simulink model "CAVE_MachE_dSPACE_250912"  (R2024a)
settings: configuration reference "ConfigSetDesktopFixedStep" (kept outside this file)
PreLoadFcn:
  | VSS_BICYCLE=Simulink.Variant('Dual=0');
  | VSS_DUAL=Simulink.Variant('Dual=1');
  | Dual=1;
  | load('DriveCycle2.mat')
PostLoadFcn:
  | if any(exist('dsrtsu_mdlpostloadfcn', 'file') ~= 0), dsrtsu_mdlpostloadfcn('Execute', bdroot); end
InitFcn:
  | , if any(exist('rtifpga_mdlclblib', 'file') ~= 0), rtifpga_mdlclblib('Init', bdroot); end,
  | , if any(exist('dsmpb_private', 'file') ~= 0), dsmpb_private('dsmpb_mdlclblib', 'Init', bdroot); end,
  | load('DriveCycle2.mat')
model workspace (MAT data in the model file):
  Gas = 0.383333333333
values from neighbouring files (symbols this model uses):
  CoastDown =     [Run_Simulink.mat]
  limitedMCT =     [Run_Simulink.mat]
  MCT =     [Run_Simulink.mat]
  pMCT =     [Run_Simulink.mat]
  RealSimPara =     [Run_Simulink.mat]
  Ref_speed = [13 13.007895099 13.015778396 13.023649891 13.031509584 13.039357475 13.047193564 13.055017851 13.062830336 13.070631019 13.0784199 13.086196979 ... (2669 elements, 2669x1)]    [Ref_speed_and_time.mat]
  Ref_time = [0 0.01 0.02 0.03 0.04 0.05 0.06 0.07 0.08 0.09 0.1 0.11 ... (2669 elements, 2669x1)]    [Ref_speed_and_time.mat]
  US06 =     [Run_Simulink.mat]
undefined symbols (not defined in the file or in its folder): AccelCmd, ActTqLF_Nm_, ActTqLR_Nm_, ActTqRF_Nm_, ActTqRR_Nm_, BattChargeLimitMaxPwr, BattChargeLimitSocBpts, BattChargeLimitTbl, BattChrgCapcty, BattDischargeLimitSocBpts, BattDischargeLimitTbl, BattDischargeMaxPwr, BattNumCellsParallel, BattNumCellsSeries, BattOpenVoltCapBpts, BattOpenVoltTbl, BattResistSocBpts, BattResistTbl, BattResistTempBpts, BrakeMaxPrs, BrakeMaxTrq, ChassisDistCg2FrontAxle, ChassisDistCg2RearAxle, ChassisVehMass, CltchCmd, DecelCmd, DiffRatio, DiscIntNeverNeededParam, EnvGravCnst, EnvPrs, EnvTemp, FuelSpecificGrav, GearCmd, h, InitStates, lgSw, MtrEffSpdBpts, MtrEffTbl, MtrEffTrqBpts, MtrPwrMax, MtrTrqMax, SteeringCmd, SupvsryCtrlRegenBrkCutOffTbl, SupvsryCtrlRegenSpdBpts, TestScnrioCycleNum, VEH
libraries: VSIGenLib x122, simulink x112, etargetslib x75, dsmpblib x55, vehdynlibtire x24, CarMaker4SL x20, autolibshared x19, vehdynlibsuspension x14, vehdynlibtirecommon x14, autolibutils x10, VsrLibWheel x8, autolibpowerinfoutils x6
(part 4 of 31)

== system CAVE_MachE_dSPACE_250912/Vehicle Under Test3/Environment ==
  Grade : Inport
  Friction : Constant  Value=ones(4,1).*1
  Ground Feedback : Subsystem  Variant=on  VariantControlMode=label  LabelModeActiveChoice=0
  Ground Z Level : Constant  Value=zeros(4,1)
  Subsystem : Subsystem
  Subsystem1 : Subsystem
      mask Display: disp('')
  Env : Outport
  wires:
  Subsystem/3(WindVel) -> Subsystem1/3(WindVel)
  Subsystem/2(EnvTemp) -> Subsystem1/2(EnvTemp)
  Subsystem/4(RoadGrade) -> Subsystem1/4(RoadGrade)
  Subsystem/1(EnvPrs) -> Subsystem1/1(EnvPrs)
  Subsystem1/1(Env) -> Env/1
  Friction/1 -> Ground Feedback/1(Friction)
  Ground Feedback/1(Ground) -> Subsystem1/5(GroundBus)  "Gnd"
  Ground Z Level/1 -> Ground Feedback/2(Ground Z Level)
  Grade/1 -> Subsystem/1(Grade)

== system CAVE_MachE_dSPACE_250912/Vehicle Under Test3/Monitor ==
  Monitor : Inport
  Calculate Fuel MPG : Subsystem  Commented=on
  Calculate Powertrain Energy : Subsystem
  Terminator : Terminator
  Terminator3 : Terminator
  wires:
  Calculate Fuel MPG/1(FuelEconMPG) -> Terminator/1  "FuelEconMpg"
  Monitor/1 -> Calculate Powertrain Energy/1(Monitor), Calculate Fuel MPG/1(Monitor)
  Calculate Powertrain Energy/1(TransEnrgyOutkWh) -> Terminator3/1  "DiffEnrgyInkWh"

== system CAVE_MachE_dSPACE_250912/Vehicle Under Test3/Performance Calculations ==
  VehSpd : Inport
  BattPwr : Inport  Port=2
  Divide : Product  Inputs=*/
  Divide1 : Product  Inputs=*/
  Divide2 : Product  Inputs=*/
  Integrator : Integrator
  Integrator1 : Integrator
  L/100 Km Calc : Product  Inputs=/*
  Product : Product
  Rate Transition3 : RateTransition  Deterministic=off
  Saturation : Saturate  UpperLimit=Inf  LowerLimit=0.001
  Saturation1 : Saturate  UpperLimit=Inf  LowerLimit=1e-3
  Sqrt : Sqrt
  US EPA kwh/USgal equivalent : Constant  Value=33.7
  US MPG Calc : Product  Inputs=*/
  m to 100Km : Gain  Gain=1/1000/100
  m to mile : Gain  Gain=0.000621371
  m^3 per gal : Gain  Gain=0.00378541
  m^3 to L : Gain  Gain=1000
  m^3 to US Gal : Gain  Gain=264.172
  s per h : Constant  Value=3600
  w per kw : Constant  Value=1000
  US MPG : Outport  VectorParamsAs1DForOutWhenUnconnected=off
  L/100Km : Outport  Port=2  VectorParamsAs1DForOutWhenUnconnected=off
  wires:
  VehSpd/1 -> Product/1, Product/2
  Product/1 -> Sqrt/1
  Sqrt/1 -> Integrator/1
  BattPwr/1 -> Divide/1
  US EPA kwh/USgal equivalent/1 -> Divide2/2
  m^3 per gal/1 -> Integrator1/1
  Divide1/1 -> m^3 per gal/1
  s per h/1 -> Divide1/2
  Divide2/1 -> Divide1/1
  Divide/1 -> Divide2/1
  w per kw/1 -> Divide/2
  Rate Transition3/1 -> US MPG/1  "US MPG"
  Saturation1/1 -> US MPG Calc/2
  US MPG Calc/1 -> Rate Transition3/1
  L/100 Km Calc/1 -> L/100Km/1  "L/100Km"
  m to 100Km/1 -> Saturation/1
  Saturation/1 -> L/100 Km Calc/1
  Integrator1/1 -> m^3 to L/1, m^3 to US Gal/1
  m to mile/1 -> US MPG Calc/1
  Integrator/1 -> m to 100Km/1, m to mile/1
  m^3 to L/1 -> L/100 Km Calc/2
  m^3 to US Gal/1 -> Saturation1/1

== system CAVE_MachE_dSPACE_250912/Vehicle Under Test3/Vehicle ==
  note: With tire radius correction of 1.14
  note: NOT USED
  note: Vehicle simulation type:
      | 0- Simulink offline model
      | 1- Rototest HIL model
  note: NOT USED
  Env : Inport
  Driver : Inport  Port=2
  CarCmd : Inport  Port=3
  Abs : Abs  Commented=on  SaturateOnIntegerOverflow=off
  Actuation and Outputs : Subsystem
  AxT : Scope
  AxT2 : Scope  Commented=on
  Battery : Subsystem
  Bus Creator : BusCreator  Inputs=6
  Bus Selector : BusSelector  OutputSignals=Omega
  Bus Selector1 : BusSelector  Commented=on  OutputSignals=BRAKE_LAMP_BOOL_CAN,STEERING_ANGLE_DEG_CAN
  Bus Selector2 : BusSelector  Commented=on  OutputSignals=CarTrqT2W,VehSpd,Fx
  Bus Selector3 : BusSelector  Commented=on  OutputSignals=PT IF WFL rotv,PT IF WFR rotv,PT IF WRL rotv,PT IF WRR rotv
  Constant : Constant  Commented=on  Value=0  SampleTime=-1
  Data Type Conversion : DataTypeConversion  Commented=on  SaturateOnIntegerOverflow=off  RndMeth=Floor
  Data Type Conversion1 : DataTypeConversion  Commented=on  SaturateOnIntegerOverflow=off  RndMeth=Floor
  DriveCycle_trigger : Constant  Value=0
  Driver and Drive Cycle : Subsystem  TreatAsAtomicUnit=on
  From CAN : Subsystem  Commented=on
  From10 : From  Commented=on  GotoTag=VehSpdKph
  Front Wheel Drive : Subsystem  Variant=on  VariantControlMode=label  VariantControl=1  LabelModeActiveChoice=Choice
  Gain : Gain  Gain=3.6
  Gain1 : Gain  Commented=on  Gain=3.6*1.1414
  Goto10 : Goto  Commented=on  GotoTag=VehSpdKph
  Goto7 : Goto  Commented=on  GotoTag=BrakePressedCAN
  Goto8 : Goto  Commented=on  GotoTag=SteeringCAN
  Motor : Subsystem
  MtT : Scope
  MtT1 : Scope
  Multiport Switch : MultiPortSwitch  DataPortOrder=Zero-based contiguous  Inputs=2  zeroidx=on  SaturateOnIntegerOverflow=off  InputSameDT=off
  "Powertrain Supervisory Controller " : Subsystem  AncestorBlock=LibPtSupervisoryCtrl/Powertrain Supervisory Controller
  "Rototest UDP RX ExternalMode  " : Subsystem  Commented=on
  "Rototest UDP TX ExternalMode  " : Subsystem  Commented=on
  Rototest and ORNL Interface : Subsystem  Commented=on
  SUMO_speed_level : Constant  Value=0
  Scope : Scope
  Switch : Switch  Commented=on  Threshold=0.1  SaturateOnIntegerOverflow=off  InputSameDT=off
  Terminator{,1..2,4} (4 alike) : Terminator  Commented=on
  Terminator3 : Terminator
  To Workspace1 : ToWorkspace  VariableName=rotoOmega1  SampleTime=-1
      settings: Save2DSignal=2-D array (concatenate along first dimension)
  To Workspace2 : ToWorkspace  Commented=on  VariableName=rotoOmega  SampleTime=-1
      settings: Save2DSignal=2-D array (concatenate along first dimension)
  Transfer Fcn{,1..3} (4 alike) : TransferFcn  Commented=on  Denominator=[0.01 1]
  Transfer Fcn12 : TransferFcn  Commented=on  Denominator=[0.02 1]
  Vector Concatenate : Concatenate  Commented=on  NumInputs=4
  Vehicle Dynamics : Subsystem  Variant=on  VariantControlMode=label  LabelModeActiveChoice=Veh14DOF  mask{VehDynSel=Vehicle 14DOF}
      mask prompts: VehDynSel "Select the driver"
      mask init: same as CAVE_MachE_dSPACE_250912/Vehicle Under Test2/Vehicle/Vehicle Dynamics
      mask TypeOptions VehDynSel: Vehicle Longitudinal | Vehicle 7DOF | Vehicle 14DOF
  VehicleSimulationType : Constant  Value=0
  omega : Scope
  Veh : Outport
  Output : Outport  Port=2
  wires:
  "Powertrain Supervisory Controller "/1(SupvsryCtrl) -> Vehicle Dynamics/2(SupvsryCtrl), Motor/1(SupvsryCtrl), [SupvsryCtrl]
  Driver/1 -> "Powertrain Supervisory Controller "/1(Driver)
  Bus Creator/1 -> Veh/1  "Veh"
  [SupvsryCtrl] -> Bus Creator/1  "SupvsryCtrl"
  [Batt] -> Bus Creator/2  "Batt"
  [Mtr] -> Bus Creator/3  "Mtr"
  [Whl] -> Bus Creator/5  "Whl"
  [Chassis] -> Bus Creator/6  "Chassis"
  Battery/1(Batt) -> [Batt], "Powertrain Supervisory Controller "/4(Batt)
  Motor/1(Mtr) -> "Powertrain Supervisory Controller "/3(Mtr), [Mtr]
  Env/1 -> Vehicle Dynamics/1(Env)
  Vehicle Dynamics/2(Chassis) -> "Powertrain Supervisory Controller "/2(Chassis), [Chassis]
  Vehicle Dynamics/1(Whl) -> [Whl]
  [Whl] -> Bus Selector/1
  [Diff] -> Bus Creator/4  "Diff"
  Front Wheel Drive/1(Diff) -> [Diff]
  Front Wheel Drive/3(PropShaftSpd) -> MtT1/1, Motor/2(MtrSpd)
  Motor/2(MtrTrq) -> Front Wheel Drive/1(DrvShfTrq), MtT/1
  Front Wheel Drive/2(AxlTrq) -> AxT/1, Vehicle Dynamics/3(AxlTrq)
  Rototest and ORNL Interface/2(Powertrain Out) -> Bus Selector3/1, Terminator/1
  Rototest and ORNL Interface/4(WhlSpd) -> To Workspace2/1, Terminator4/1  "WhlSpdCmd"
  Vehicle Dynamics/3(RototestInput) -> [RototestInput]
  VehicleSimulationType/1 -> Multiport Switch/1
  Driver and Drive Cycle/1(DriverBus) -> Actuation and Outputs/1(Driver Commands)
  Bus Selector1/1 -> Data Type Conversion1/1  "<BRAKE_LAMP_BOOL_CAN>"
  Data Type Conversion/1 -> Goto8/1  "SteerAngleCAN"
  "Rototest UDP RX ExternalMode  "/1(Data Vector) -> Rototest and ORNL Interface/2(UDP Input)
  Data Type Conversion1/1 -> Rototest and ORNL Interface/3(BRAKE_PRESSED), Goto7/1, Terminator2/1  "BrakePressed_flag"
  Bus Selector1/2 -> Data Type Conversion/1  "<STEERING_ANGLE_DEG_CAN>"
  From CAN/1(IO_Out) -> Bus Selector1/1
  Actuation and Outputs/1(BrakeSwitch) -> From CAN/1(BrakeSwitch)
  Actuation and Outputs/2(CAVE_Driver) -> Terminator3/1  "CAVE_Driver_Cmd"
  Rototest and ORNL Interface/3(DataSend) -> "Rototest UDP TX ExternalMode  "/1(Rototest_UDP_TX)  "Rototest_UDP_TX"
  Rototest and ORNL Interface/1(BrakeUpd) -> Terminator1/1
  [RototestInput] -> Bus Selector2/1
  Bus Selector2/3 -> Rototest and ORNL Interface/5(FXIN)  "<Fx>"
  Bus Selector2/2 -> Transfer Fcn12/1  "<VehSpd>"
  Bus Selector2/1 -> Rototest and ORNL Interface/1(CarTrqT2W)  "<CarTrqT2W>"
  Bus Selector/1 -> Multiport Switch/2  "<Omega>"
  Bus Selector3/1 -> Transfer Fcn/1  "<PT IF WFL rotv>"
  Bus Selector3/2 -> Transfer Fcn1/1  "<PT IF WFR rotv>"
  Bus Selector3/3 -> Transfer Fcn2/1  "<PT IF WRL rotv>"
  Bus Selector3/4 -> Transfer Fcn3/1  "<PT IF WRR rotv>"
  Vector Concatenate/1 -> Scope/1, To Workspace1/1, [OmegaRoto]
  [OmegaRoto] -> Multiport Switch/3
  Gain1/1 -> AxT2/1, Rototest and ORNL Interface/4(vehSpeedKph), Goto10/1  "VehSpdKph"
  Gain/1 -> Driver and Drive Cycle/1(Veh speed feedback [kph])
  DriveCycle_trigger/1 -> Driver and Drive Cycle/2(Veh speed cycle trigger)
  Multiport Switch/1 -> Front Wheel Drive/2(Omega), omega/1
  Constant/1 -> Switch/3
  Switch/1 -> Gain1/1
  Abs/1 -> Switch/2
  Transfer Fcn/1 -> Vector Concatenate/1
  Transfer Fcn1/1 -> Vector Concatenate/2
  Transfer Fcn2/1 -> Vector Concatenate/3
  Transfer Fcn3/1 -> Vector Concatenate/4
  Transfer Fcn12/1 -> Switch/1, Abs/1
  CarCmd/1 -> Actuation and Outputs/2(CarlaGBS), Driver and Drive Cycle/4(CarlaRef)
  Driver and Drive Cycle/2(Output) -> Output/1
  SUMO_speed_level/1 -> Driver and Drive Cycle/3(SUMO Veh speed Cmd Level)
  [vehSpeedSim] -> Gain/1
  connections:
  Battery/RConn1 -- Motor/LConn1

== system CAVE_MachE_dSPACE_250912/FIXS/RealSim Core/RealSim CreatBus ==
  In : Inport
  speedDesired : Inport  Port=2
  color : Inport  Port=3
  accelerationDesired : Inport  Port=4
  activeLaneChange : Inport  Port=5
  Bus Creator2 : BusCreator  Inputs=36  OutDataTypeStr=Bus: VehDataBus
  Bus Selector1 : BusSelector  OutputSignals=id,idLength,type,typeLength,vehicleClass,vehicleClassLength,speed,acceleration,positionX,positionY,positionZ,heading,color,linkId,linkIdLength,laneId,distanceTravel,speedDesired,accelerationDesired,hasPrecedingVehicle,precedingVehicleId,precedingVehicleIdLength,precedingVehicleDistance,precedingVehicleSpeed,signalLightId,signalLightIdLength,signalLightHeadId,signalLightDistance,signalLightColor,speedLimit,speedLimitNext,speedLimitChangeDistance,linkIdNext,linkIdNextLength,grade,activeLaneChange
  Terminator{4..7} (4 alike) : Terminator
  rgba2uint : Subsystem
  Out : Outport
  wires:
  Bus Creator2/1 -> Out/1
  rgba2uint/1(Out1) -> Bus Creator2/13  "color"
  color/1 -> rgba2uint/1(In1)  "color"
  accelerationDesired/1 -> Bus Creator2/19  "accelerationDesired"
  speedDesired/1 -> Bus Creator2/18  "speedDesired"
  activeLaneChange/1 -> Bus Creator2/36  "activeLaneChange"
  Bus Selector1/36 -> Terminator7/1  "<activeLaneChange>"
  Bus Selector1/35 -> Bus Creator2/35  "<grade>"
  Bus Selector1/34 -> Bus Creator2/34  "<linkIdNextLength>"
  Bus Selector1/33 -> Bus Creator2/33  "<linkIdNext>"
  Bus Selector1/32 -> Bus Creator2/32  "<speedLimitChangeDistance>"
  Bus Selector1/31 -> Bus Creator2/31  "<speedLimitNext>"
  Bus Selector1/30 -> Bus Creator2/30  "<speedLimit>"
  Bus Selector1/29 -> Bus Creator2/29  "<signalLightColor>"
  Bus Selector1/28 -> Bus Creator2/28  "<signalLightDistance>"
  Bus Selector1/27 -> Bus Creator2/27  "<signalLightHeadId>"
  Bus Selector1/26 -> Bus Creator2/26  "<signalLightIdLength>"
  Bus Selector1/25 -> Bus Creator2/25  "<signalLightId>"
  Bus Selector1/24 -> Bus Creator2/24  "<precedingVehicleSpeed>"
  Bus Selector1/23 -> Bus Creator2/23  "<precedingVehicleDistance>"
  Bus Selector1/22 -> Bus Creator2/22  "<precedingVehicleIdLength>"
  Bus Selector1/21 -> Bus Creator2/21  "<precedingVehicleId>"
  Bus Selector1/20 -> Bus Creator2/20  "<hasPrecedingVehicle>"
  Bus Selector1/19 -> Terminator6/1  "<accelerationDesired>"
  Bus Selector1/18 -> Terminator4/1  "<speedDesired>"
  Bus Selector1/17 -> Bus Creator2/17  "<distanceTravel>"
  Bus Selector1/16 -> Bus Creator2/16  "<laneId>"
  Bus Selector1/15 -> Bus Creator2/15  "<linkIdLength>"
  Bus Selector1/14 -> Bus Creator2/14  "<linkId>"
  Bus Selector1/13 -> Terminator5/1  "<color>"
  Bus Selector1/12 -> Bus Creator2/12  "<heading>"
  Bus Selector1/11 -> Bus Creator2/11  "<positionZ>"
  Bus Selector1/10 -> Bus Creator2/10  "<positionY>"
  Bus Selector1/9 -> Bus Creator2/9  "<positionX>"
  Bus Selector1/8 -> Bus Creator2/8  "<acceleration>"
  Bus Selector1/7 -> Bus Creator2/7  "<speed>"
  Bus Selector1/6 -> Bus Creator2/6  "<vehicleClassLength>"
  Bus Selector1/5 -> Bus Creator2/5  "<vehicleClass>"
  Bus Selector1/4 -> Bus Creator2/4  "<typeLength>"
  Bus Selector1/3 -> Bus Creator2/3  "<type>"
  Bus Selector1/2 -> Bus Creator2/2  "<idLength>"
  Bus Selector1/1 -> Bus Creator2/1  "<id>"
  In/1 -> Bus Selector1/1

== system CAVE_MachE_dSPACE_250912/FIXS/RealSim Core/dSPACE TCP In ==
  Data Type Conversion1 : DataTypeConversion  OutDataTypeStr=uint8  SaturateOnIntegerOverflow=off  RndMeth=Floor
  Data Type Conversion4 : DataTypeConversion  OutDataTypeStr=double  SaturateOnIntegerOverflow=off  RndMeth=Floor
  Display7 : Display
  Ethernet Setup : dsmpblib/Data Inport  Priority=10000
      settings: SourceProductName=dSPACE Model Interface Package for Simulink (MIPS)
  Receive_In [TCP (1)] : dsmpblib/Data Inport  Priority=10000
      settings: SourceProductName=dSPACE Model Interface Package for Simulink (MIPS)
  Receive_Out [TCP (1)] : dsmpblib/Data Outport  Priority=-10000
      settings: SourceProductName=dSPACE Model Interface Package for Simulink (MIPS)
  Status/Control_In [TCP (1)] : dsmpblib/Data Inport  Priority=10000
      settings: SourceProductName=dSPACE Model Interface Package for Simulink (MIPS)
  Terminator{19,25..27} (4 alike) : Terminator
  Transmit_In [TCP (1)] : dsmpblib/Data Inport  Priority=10000
      settings: SourceProductName=dSPACE Model Interface Package for Simulink (MIPS)
  ByteData : Outport
  nByte : Outport  Port=2
  ConnectionState : Outport  Port=3
  wires:
  Data Type Conversion4/1 -> ConnectionState/1  "ConnectionState"
  Status/Control_In [TCP (1)]/1 -> Data Type Conversion4/1  "Connection_State"
  Receive_In [TCP (1)]/4 -> Receive_Out [TCP (1)]/1
  Ethernet Setup/1 -> Terminator26/1
  Receive_In [TCP (1)]/1 -> Data Type Conversion1/1
  Transmit_In [TCP (1)]/2 -> Terminator19/1
  Transmit_In [TCP (1)]/1 -> Terminator27/1
  Receive_In [TCP (1)]/2 -> Terminator25/1
  Receive_In [TCP (1)]/3 -> nByte/1, Display7/1
  Data Type Conversion1/1 -> ByteData/1

== system CAVE_MachE_dSPACE_250912/FIXS/RealSim Core/dSPACE TCP Out ==
  ByteSend : Inport
  nMsgSend : Inport  Port=2
  sendTrigger : Inport  Port=3
  Constant : Constant
  Constant1 : Constant  Value=0
  Data Type Conversion : DataTypeConversion  SaturateOnIntegerOverflow=off  RndMeth=Floor
  Data Type Conversion4 : DataTypeConversion  SaturateOnIntegerOverflow=off  RndMeth=Floor
  Display7 : Display
  Transmit_Out [TCP (1)] : dsmpblib/Data Outport  Priority=-10000
      settings: SourceProductName=dSPACE Model Interface Package for Simulink (MIPS)
  switch for 0.1 send out : Switch  Criteria=u2 > Threshold  SaturateOnIntegerOverflow=off  InputSameDT=off
  wires:
  Constant1/1 -> switch for 0.1 send out/3
  nMsgSend/1 -> Data Type Conversion4/1
  Data Type Conversion4/1 -> switch for 0.1 send out/1, Display7/1
  switch for 0.1 send out/1 -> Transmit_Out [TCP (1)]/2  "sendByteSize_RealSimPack"
  sendTrigger/1 -> switch for 0.1 send out/2
  Constant/1 -> Data Type Conversion/1
  Data Type Conversion/1 -> Transmit_Out [TCP (1)]/3
  ByteSend/1 -> Transmit_Out [TCP (1)]/1

== system CAVE_MachE_dSPACE_250912/FIXS/RealSim Core/speedCmd_gen ==
  speedIn : Inport
  initSpeed : Inport  Port=2
  connectionState : Inport  Port=3
  tIn : Inport  Port=4
  Add : Sum  Inputs=+-
  Compare To Constant : simulink/Logic and Bit Operations/Compare To Constant  relop=>  const=0  OutDataTypeStr=boolean
  Compare To Zero : simulink/Logic and Bit Operations/Compare To Zero  relop===  OutDataTypeStr=boolean
  Constant2 : Constant  Value=3
  Logical Operator : Logic  AllPortsSameDT=off  OutDataTypeStr=boolean
  Switch1 : Switch  Criteria=u2 ~= 0  SaturateOnIntegerOverflow=off  InputSameDT=off
  speedCmd : Outport
  wires:
  Add/1 -> Compare To Zero/1
  initSpeed/1 -> Switch1/3
  Constant2/1 -> Add/2
  Switch1/1 -> speedCmd/1
  connectionState/1 -> Add/1  "connectionState"
  speedIn/1 -> Switch1/1
  tIn/1 -> Compare To Constant/1  "tIn"
  Compare To Constant/1 -> Logical Operator/2
  Logical Operator/1 -> Switch1/2
  Compare To Zero/1 -> Logical Operator/1

== system CAVE_MachE_dSPACE_250912/FIXS1/RealSim Core/Subsystem ==
  speedIn : Inport
  initSpeed : Inport  Port=2
  connectionState : Inport  Port=3
  tIn : Inport  Port=4
  Add : Sum  Inputs=+-
  Compare To Constant : simulink/Logic and Bit Operations/Compare To Constant  relop=>  const=0  OutDataTypeStr=boolean
  Compare To Zero : simulink/Logic and Bit Operations/Compare To Zero  relop===  OutDataTypeStr=boolean
  Constant2 : Constant  Value=3
  Logical Operator : Logic  AllPortsSameDT=off  OutDataTypeStr=boolean
  Switch1 : Switch  Criteria=u2 ~= 0  SaturateOnIntegerOverflow=off  InputSameDT=off
  speedCmd : Outport
  wires:
  Add/1 -> Compare To Zero/1
  initSpeed/1 -> Switch1/3
  Constant2/1 -> Add/2
  Switch1/1 -> speedCmd/1
  connectionState/1 -> Add/1  "connectionState"
  speedIn/1 -> Switch1/1
  tIn/1 -> Compare To Constant/1  "tIn"
  Compare To Constant/1 -> Logical Operator/2
  Logical Operator/1 -> Switch1/2
  Compare To Zero/1 -> Logical Operator/1

== system CAVE_MachE_dSPACE_250912/FIXS1/RealSim Core/dSPACE TCP In ==
  Data Type Conversion1 : DataTypeConversion  OutDataTypeStr=uint8  SaturateOnIntegerOverflow=off  RndMeth=Floor
  Data Type Conversion4 : DataTypeConversion  OutDataTypeStr=double  SaturateOnIntegerOverflow=off  RndMeth=Floor
  Display7 : Display
  Ethernet Setup (1) : dsmpblib/Data Inport  Priority=10000
      settings: SourceProductName=dSPACE Model Interface Package for Simulink (MIPS)
  Receive [TCP (1)] : dsmpblib/Data Inport  Priority=10000
      settings: SourceProductName=dSPACE Model Interface Package for Simulink (MIPS)
  Receive_Out [TCP (1)] : dsmpblib/Data Outport  Priority=-10000
      settings: SourceProductName=dSPACE Model Interface Package for Simulink (MIPS)
  Status/Control_In [TCP (1)] : dsmpblib/Data Inport  Priority=10000
      settings: SourceProductName=dSPACE Model Interface Package for Simulink (MIPS)
  Terminator{19,25..27} (4 alike) : Terminator
  Transmit_In [TCP (1)] : dsmpblib/Data Inport  Priority=10000
      settings: SourceProductName=dSPACE Model Interface Package for Simulink (MIPS)
  ByteData : Outport
  nByte : Outport  Port=2
  ConnectionState : Outport  Port=3
  wires:
  Data Type Conversion4/1 -> ConnectionState/1  "ConnectionState"
  Status/Control_In [TCP (1)]/1 -> Data Type Conversion4/1  "Connection_State"
  ? -> Receive_Out [TCP (1)]/1
  Ethernet Setup (1)/1 -> Terminator26/1
  Receive [TCP (1)]/1 -> Data Type Conversion1/1
  ? -> Terminator19/1
  Transmit_In [TCP (1)]/1 -> Terminator27/1
  ? -> Terminator25/1
  ? -> Display7/1, nByte/1
  Data Type Conversion1/1 -> ByteData/1

== system CAVE_MachE_dSPACE_250912/FIXS1/RealSim Core/dSPACE TCP Out ==
  ByteSend : Inport
  nMsgSend : Inport  Port=2
  sendTrigger : Inport  Port=3
  Constant : Constant
  Constant1 : Constant  Value=0
  Data Type Conversion : DataTypeConversion  SaturateOnIntegerOverflow=off  RndMeth=Floor
  Data Type Conversion4 : DataTypeConversion  SaturateOnIntegerOverflow=off  RndMeth=Floor
  Display7 : Display
  Transmit_Out [TCP (1)] : dsmpblib/Data Outport  Priority=-10000
      settings: SourceProductName=dSPACE Model Interface Package for Simulink (MIPS)
  switch for 0.1 send out : Switch  Criteria=u2 > Threshold  SaturateOnIntegerOverflow=off  InputSameDT=off
  wires:
  Constant1/1 -> switch for 0.1 send out/3
  nMsgSend/1 -> Data Type Conversion4/1
  Data Type Conversion4/1 -> switch for 0.1 send out/1, Display7/1
  switch for 0.1 send out/1 -> ?  "sendByteSize_RealSimPack"
  ByteSend/1 -> Transmit_Out [TCP (1)]/1
  sendTrigger/1 -> switch for 0.1 send out/2
  Constant/1 -> Data Type Conversion/1
  Data Type Conversion/1 -> ?

== system CAVE_MachE_dSPACE_250912/FIXS1/RealSim Translate CM Signal to Bus as Feedback to SUMO//VISSIM/RealSim CreatBus ==
  VehDataBusIn : Inport
  speedDesired : Inport  Port=2
  color : Inport  Port=3
  accelerationDesired : Inport  Port=4
  activeLaneChange : Inport  Port=5
  positionX : Inport  Port=6
  Bus Creator2 : BusCreator  Inputs=36  OutDataTypeStr=Bus: VehDataBus
  Bus Selector1 : BusSelector  OutputSignals=id,idLength,type,typeLength,vehicleClass,vehicleClassLength,speed,acceleration,positionX,positionY,positionZ,heading,color,linkId,linkIdLength,laneId,distanceTravel,speedDesired,accelerationDesired,hasPrecedingVehicle,precedingVehicleId,precedingVehicleIdLength,precedingVehicleDistance,precedingVehicleSpeed,signalLightId,signalLightIdLength,signalLightHeadId,signalLightDistance,signalLightColor,speedLimit,speedLimitNext,speedLimitChangeDistance,linkIdNext,linkIdNextLength,grade,activeLaneChange
  Terminator{1,4..7} (5 alike) : Terminator
  rgba2uint : Subsystem
  Out : Outport
  wires:
  VehDataBusIn/1 -> Bus Selector1/1
  Bus Selector1/1 -> Bus Creator2/1  "<id>"
  Bus Selector1/2 -> Bus Creator2/2  "<idLength>"
  Bus Selector1/3 -> Bus Creator2/3  "<type>"
  Bus Selector1/4 -> Bus Creator2/4  "<typeLength>"
  Bus Selector1/5 -> Bus Creator2/5  "<vehicleClass>"
  Bus Selector1/6 -> Bus Creator2/6  "<vehicleClassLength>"
  Bus Selector1/7 -> Bus Creator2/7  "<speed>"
  Bus Selector1/8 -> Bus Creator2/8  "<acceleration>"
  Bus Selector1/9 -> Terminator1/1  "<positionX>"
  Bus Selector1/10 -> Bus Creator2/10  "<positionY>"
  Bus Selector1/11 -> Bus Creator2/11  "<positionZ>"
  Bus Selector1/12 -> Bus Creator2/12  "<heading>"
  Bus Selector1/13 -> Terminator5/1  "<color>"
  Bus Selector1/14 -> Bus Creator2/14  "<linkId>"
  Bus Selector1/15 -> Bus Creator2/15  "<linkIdLength>"
  Bus Selector1/16 -> Bus Creator2/16  "<laneId>"
  Bus Selector1/17 -> Bus Creator2/17  "<distanceTravel>"
  Bus Selector1/18 -> Terminator4/1  "<speedDesired>"
  Bus Selector1/19 -> Terminator6/1  "<accelerationDesired>"
  Bus Selector1/20 -> Bus Creator2/20  "<hasPrecedingVehicle>"
  Bus Selector1/21 -> Bus Creator2/21  "<precedingVehicleId>"
  Bus Selector1/22 -> Bus Creator2/22  "<precedingVehicleIdLength>"
  Bus Selector1/23 -> Bus Creator2/23  "<precedingVehicleDistance>"
  Bus Selector1/24 -> Bus Creator2/24  "<precedingVehicleSpeed>"
  Bus Selector1/25 -> Bus Creator2/25  "<signalLightId>"
  Bus Selector1/26 -> Bus Creator2/26  "<signalLightIdLength>"
  Bus Selector1/27 -> Bus Creator2/27  "<signalLightHeadId>"
  Bus Selector1/28 -> Bus Creator2/28  "<signalLightDistance>"
  Bus Selector1/29 -> Bus Creator2/29  "<signalLightColor>"
  Bus Selector1/30 -> Bus Creator2/30  "<speedLimit>"
  Bus Selector1/31 -> Bus Creator2/31  "<speedLimitNext>"
  Bus Selector1/32 -> Bus Creator2/32  "<speedLimitChangeDistance>"
  Bus Selector1/33 -> Bus Creator2/33  "<linkIdNext>"
  Bus Selector1/34 -> Bus Creator2/34  "<linkIdNextLength>"
  Bus Selector1/35 -> Bus Creator2/35  "<grade>"
  Bus Selector1/36 -> Terminator7/1  "<activeLaneChange>"
  activeLaneChange/1 -> Bus Creator2/36  "activeLaneChange"
  speedDesired/1 -> Bus Creator2/18  "speedDesired"
  accelerationDesired/1 -> Bus Creator2/19  "accelerationDesired"
  color/1 -> rgba2uint/1(In1)  "color"
  rgba2uint/1(Out1) -> Bus Creator2/13  "color"
  Bus Creator2/1 -> Out/1
  positionX/1 -> Bus Creator2/9  "positionX"

== system CAVE_MachE_dSPACE_250912/FIXS1/RealSim Translate CM Signal to Bus as Feedback to SUMO//VISSIM/RealSim CreatBus2 ==
  note: activeLaneChange is set more for VISSIM co-simulation
  In : Inport
  positionX : Inport  Port=2
  positionY : Inport  Port=3
  positionZ : Inport  Port=4
  heading : Inport  Port=5
  color : Inport  Port=6
  speedDesired : Inport  Port=7
  speedDesired1 : Inport  Port=8
  Bus Creator1 : BusCreator  Inputs=36  OutDataTypeStr=Bus: VehDataBus
  Bus Selector1 : BusSelector  OutputSignals=id,idLength,type,typeLength,vehicleClass,vehicleClassLength,speed,acceleration,positionX,positionY,positionZ,heading,color,linkId,linkIdLength,laneId,distanceTravel,speedDesired,accelerationDesired,hasPrecedingVehicle,precedingVehicleId,precedingVehicleIdLength,precedingVehicleDistance,precedingVehicleSpeed,signalLightId,signalLightIdLength,signalLightHeadId,signalLightDistance,signalLightColor,speedLimit,speedLimitNext,speedLimitChangeDistance,linkIdNext,linkIdNextLength,grade,activeLaneChange
  Terminator{,1..7} (8 alike) : Terminator
  activeLaneChange : Constant  Value=0
  Out : Outport
  wires:
  Bus Selector1/1 -> Bus Creator1/1  "<id>"
  Bus Selector1/2 -> Bus Creator1/2  "<idLength>"
  Bus Selector1/3 -> Bus Creator1/3  "<type>"
  Bus Selector1/4 -> Bus Creator1/4  "<typeLength>"
  Bus Selector1/5 -> Bus Creator1/5  "<vehicleClass>"
  Bus Selector1/6 -> Bus Creator1/6  "<vehicleClassLength>"
  Bus Selector1/7 -> Bus Creator1/7  "<speed>"
  Bus Selector1/8 -> Bus Creator1/8  "<acceleration>"
  Bus Selector1/9 -> Terminator6/1  "<positionX>"
  Bus Selector1/10 -> Terminator5/1  "<positionY>"
  Bus Selector1/11 -> Terminator4/1  "<positionZ>"
  Bus Selector1/12 -> Terminator1/1  "<heading>"
  Bus Selector1/13 -> Terminator3/1  "<color>"
  Bus Selector1/14 -> Bus Creator1/14  "<linkId>"
  Bus Selector1/15 -> Bus Creator1/15  "<linkIdLength>"
  Bus Selector1/16 -> Bus Creator1/16  "<laneId>"
  Bus Selector1/17 -> Bus Creator1/17  "<distanceTravel>"
  Bus Selector1/18 -> Terminator2/1  "<speedDesired>"
  Bus Selector1/19 -> Terminator7/1  "<accelerationDesired>"
  Bus Selector1/20 -> Bus Creator1/20  "<hasPrecedingVehicle>"
  Bus Selector1/21 -> Bus Creator1/21  "<precedingVehicleId>"
  Bus Selector1/22 -> Bus Creator1/22  "<precedingVehicleIdLength>"
  Bus Selector1/23 -> Bus Creator1/23  "<precedingVehicleDistance>"
  Bus Selector1/24 -> Bus Creator1/24  "<precedingVehicleSpeed>"
  Bus Selector1/25 -> Bus Creator1/25  "<signalLightId>"
  Bus Selector1/26 -> Bus Creator1/26  "<signalLightIdLength>"
  Bus Selector1/27 -> Bus Creator1/27  "<signalLightHeadId>"
  Bus Selector1/28 -> Bus Creator1/28  "<signalLightDistance>"
  Bus Selector1/29 -> Bus Creator1/29  "<signalLightColor>"
  Bus Selector1/30 -> Bus Creator1/30  "<speedLimit>"
  Bus Selector1/31 -> Bus Creator1/31  "<speedLimitNext>"
  Bus Selector1/32 -> Bus Creator1/32  "<speedLimitChangeDistance>"
  Bus Selector1/33 -> Bus Creator1/33  "<linkIdNext>"
  Bus Selector1/34 -> Bus Creator1/34  "<linkIdNextLength>"
  Bus Selector1/36 -> Terminator/1  "<activeLaneChange>"
  positionY/1 -> Bus Creator1/10  "positionY"
  heading/1 -> Bus Creator1/12  "heading"
  color/1 -> Bus Creator1/13  "color"
  positionX/1 -> Bus Creator1/9  "positionX"
  speedDesired/1 -> Bus Creator1/18  "speedDesired"
  positionZ/1 -> Bus Creator1/11  "positionZ"
  Bus Creator1/1 -> Out/1
  In/1 -> Bus Selector1/1
  activeLaneChange/1 -> Bus Creator1/36  "activeLaneChange"
  Bus Selector1/35 -> Bus Creator1/35  "<grade>"
  speedDesired1/1 -> Bus Creator1/19  "speedDesired"

== system CAVE_MachE_dSPACE_250912/RealSim1/ToRealSim/RealSim CreatBus ==
  In : Inport
  speedDesired : Inport  Port=2
  color : Inport  Port=3
  accelerationDesired : Inport  Port=4
  activeLaneChange : Inport  Port=5
  Bus Creator2 : BusCreator  Inputs=36  OutDataTypeStr=Bus: VehDataBus
  Bus Selector1 : BusSelector  OutputSignals=id,idLength,type,typeLength,vehicleClass,vehicleClassLength,speed,acceleration,positionX,positionY,positionZ,heading,color,linkId,linkIdLength,laneId,distanceTravel,speedDesired,accelerationDesired,hasPrecedingVehicle,precedingVehicleId,precedingVehicleIdLength,precedingVehicleDistance,precedingVehicleSpeed,signalLightId,signalLightIdLength,signalLightHeadId,signalLightDistance,signalLightColor,speedLimit,speedLimitNext,speedLimitChangeDistance,linkIdNext,linkIdNextLength,grade,activeLaneChange
  Terminator{4..7} (4 alike) : Terminator
  rgba2uint : Subsystem
  Out : Outport
  wires:
  Bus Creator2/1 -> Out/1
  rgba2uint/1(Out1) -> Bus Creator2/13  "color"
  color/1 -> rgba2uint/1(In1)  "color"
  accelerationDesired/1 -> Bus Creator2/19  "accelerationDesired"
  speedDesired/1 -> Bus Creator2/18  "speedDesired"
  activeLaneChange/1 -> Bus Creator2/36  "activeLaneChange"
  Bus Selector1/36 -> Terminator7/1  "<activeLaneChange>"
  Bus Selector1/35 -> Bus Creator2/35  "<grade>"
  Bus Selector1/34 -> Bus Creator2/34  "<linkIdNextLength>"
  Bus Selector1/33 -> Bus Creator2/33  "<linkIdNext>"
  Bus Selector1/32 -> Bus Creator2/32  "<speedLimitChangeDistance>"
  Bus Selector1/31 -> Bus Creator2/31  "<speedLimitNext>"
  Bus Selector1/30 -> Bus Creator2/30  "<speedLimit>"
  Bus Selector1/29 -> Bus Creator2/29  "<signalLightColor>"
  Bus Selector1/28 -> Bus Creator2/28  "<signalLightDistance>"
  Bus Selector1/27 -> Bus Creator2/27  "<signalLightHeadId>"
  Bus Selector1/26 -> Bus Creator2/26  "<signalLightIdLength>"
  Bus Selector1/25 -> Bus Creator2/25  "<signalLightId>"
  Bus Selector1/24 -> Bus Creator2/24  "<precedingVehicleSpeed>"
  Bus Selector1/23 -> Bus Creator2/23  "<precedingVehicleDistance>"
  Bus Selector1/22 -> Bus Creator2/22  "<precedingVehicleIdLength>"
  Bus Selector1/21 -> Bus Creator2/21  "<precedingVehicleId>"
  Bus Selector1/20 -> Bus Creator2/20  "<hasPrecedingVehicle>"
  Bus Selector1/19 -> Terminator6/1  "<accelerationDesired>"
  Bus Selector1/18 -> Terminator4/1  "<speedDesired>"
  Bus Selector1/17 -> Bus Creator2/17  "<distanceTravel>"
  Bus Selector1/16 -> Bus Creator2/16  "<laneId>"
  Bus Selector1/15 -> Bus Creator2/15  "<linkIdLength>"
  Bus Selector1/14 -> Bus Creator2/14  "<linkId>"
  Bus Selector1/13 -> Terminator5/1  "<color>"
  Bus Selector1/12 -> Bus Creator2/12  "<heading>"
  Bus Selector1/11 -> Bus Creator2/11  "<positionZ>"
  Bus Selector1/10 -> Bus Creator2/10  "<positionY>"
  Bus Selector1/9 -> Bus Creator2/9  "<positionX>"
  Bus Selector1/8 -> Bus Creator2/8  "<acceleration>"
  Bus Selector1/7 -> Bus Creator2/7  "<speed>"
  Bus Selector1/6 -> Bus Creator2/6  "<vehicleClassLength>"
  Bus Selector1/5 -> Bus Creator2/5  "<vehicleClass>"
  Bus Selector1/4 -> Bus Creator2/4  "<typeLength>"
  Bus Selector1/3 -> Bus Creator2/3  "<type>"
  Bus Selector1/2 -> Bus Creator2/2  "<idLength>"
  Bus Selector1/1 -> Bus Creator2/1  "<id>"
  In/1 -> Bus Selector1/1

== system CAVE_MachE_dSPACE_250912/RealSim2/ToRealSim/RealSim CreatBus ==
  In : Inport
  speedDesired : Inport  Port=2
  color : Inport  Port=3
  accelerationDesired : Inport  Port=4
  activeLaneChange : Inport  Port=5
  Bus Creator2 : BusCreator  Inputs=36  OutDataTypeStr=Bus: VehDataBus
  Bus Selector1 : BusSelector  OutputSignals=id,idLength,type,typeLength,vehicleClass,vehicleClassLength,speed,acceleration,positionX,positionY,positionZ,heading,color,linkId,linkIdLength,laneId,distanceTravel,speedDesired,accelerationDesired,hasPrecedingVehicle,precedingVehicleId,precedingVehicleIdLength,precedingVehicleDistance,precedingVehicleSpeed,signalLightId,signalLightIdLength,signalLightHeadId,signalLightDistance,signalLightColor,speedLimit,speedLimitNext,speedLimitChangeDistance,linkIdNext,linkIdNextLength,grade,activeLaneChange
  Terminator{4..7} (4 alike) : Terminator
  rgba2uint : Subsystem
  Out : Outport
  wires:
  In/1 -> Bus Selector1/1
  Bus Selector1/1 -> Bus Creator2/1  "<id>"
  Bus Selector1/2 -> Bus Creator2/2  "<idLength>"
  Bus Selector1/3 -> Bus Creator2/3  "<type>"
  Bus Selector1/4 -> Bus Creator2/4  "<typeLength>"
  Bus Selector1/5 -> Bus Creator2/5  "<vehicleClass>"
  Bus Selector1/6 -> Bus Creator2/6  "<vehicleClassLength>"
  Bus Selector1/7 -> Bus Creator2/7  "<speed>"
  Bus Selector1/8 -> Bus Creator2/8  "<acceleration>"
  Bus Selector1/9 -> Bus Creator2/9  "<positionX>"
  Bus Selector1/10 -> Bus Creator2/10  "<positionY>"
  Bus Selector1/11 -> Bus Creator2/11  "<positionZ>"
  Bus Selector1/12 -> Bus Creator2/12  "<heading>"
  Bus Selector1/13 -> Terminator5/1  "<color>"
  Bus Selector1/14 -> Bus Creator2/14  "<linkId>"
  Bus Selector1/15 -> Bus Creator2/15  "<linkIdLength>"
  Bus Selector1/16 -> Bus Creator2/16  "<laneId>"
  Bus Selector1/17 -> Bus Creator2/17  "<distanceTravel>"
  Bus Selector1/18 -> Terminator4/1  "<speedDesired>"
  Bus Selector1/19 -> Terminator6/1  "<accelerationDesired>"
  Bus Selector1/20 -> Bus Creator2/20  "<hasPrecedingVehicle>"
  Bus Selector1/21 -> Bus Creator2/21  "<precedingVehicleId>"
  Bus Selector1/22 -> Bus Creator2/22  "<precedingVehicleIdLength>"
  Bus Selector1/23 -> Bus Creator2/23  "<precedingVehicleDistance>"
  Bus Selector1/24 -> Bus Creator2/24  "<precedingVehicleSpeed>"
  Bus Selector1/25 -> Bus Creator2/25  "<signalLightId>"
  Bus Selector1/26 -> Bus Creator2/26  "<signalLightIdLength>"
  Bus Selector1/27 -> Bus Creator2/27  "<signalLightHeadId>"
  Bus Selector1/28 -> Bus Creator2/28  "<signalLightDistance>"
  Bus Selector1/29 -> Bus Creator2/29  "<signalLightColor>"
  Bus Selector1/30 -> Bus Creator2/30  "<speedLimit>"
  Bus Selector1/31 -> Bus Creator2/31  "<speedLimitNext>"
  Bus Selector1/32 -> Bus Creator2/32  "<speedLimitChangeDistance>"
  Bus Selector1/33 -> Bus Creator2/33  "<linkIdNext>"
  Bus Selector1/34 -> Bus Creator2/34  "<linkIdNextLength>"
  Bus Selector1/35 -> Bus Creator2/35  "<grade>"
  Bus Selector1/36 -> Terminator7/1  "<activeLaneChange>"
  activeLaneChange/1 -> Bus Creator2/36  "activeLaneChange"
  speedDesired/1 -> Bus Creator2/18  "speedDesired"
  accelerationDesired/1 -> Bus Creator2/19  "accelerationDesired"
  color/1 -> rgba2uint/1(In1)  "color"
  rgba2uint/1(Out1) -> Bus Creator2/13  "color"
  Bus Creator2/1 -> Out/1

== system CAVE_MachE_dSPACE_250912/Vehicle Under Test2/Environment/Ground Feedback ==
  note: 1) Add Subsystem or Model blocks as valid variant choices.
      | 2) You cannot connect blocks at this level. At simulation, connectivity is automatically
      | determined, based on the active variant and port name matching.
  Friction : Inport
  Ground Z Level : Inport  Port=2
  3D Engine : Subsystem  VariantControl=1
  Constant : Subsystem  VariantControl=0
  Ground : Outport  VectorParamsAs1DForOutWhenUnconnected=off

== system CAVE_MachE_dSPACE_250912/Vehicle Under Test2/Environment/Subsystem ==
  Grade : Inport
  Constant : Constant  Value=EnvPrs
  Constant1 : Constant  Value=EnvTemp
  Constant2 : Constant  Value=0
  Constant3 : Constant  Value=0
  Constant4 : Constant  Value=0
  Signal Specification : SignalSpecification  Unit=Pa
  Signal Specification1 : SignalSpecification  Unit=K
  Signal Specification2 : SignalSpecification  Unit=rad
  Signal Specification3 : SignalSpecification  Unit=m/s
  Signal Specification4 : SignalSpecification  Unit=m/s
  Signal Specification5 : SignalSpecification  Unit=m/s
  Vector Concatenate : Concatenate  NumInputs=3
  EnvPrs : Outport
  EnvTemp : Outport  Port=2
  WindVel : Outport  Port=3
  RoadGrade : Outport  Port=4
  wires:
  Constant/1 -> Signal Specification/1
  Constant2/1 -> Signal Specification3/1
  Constant1/1 -> Signal Specification1/1
  Grade/1 -> Signal Specification2/1
  Signal Specification/1 -> EnvPrs/1
  Signal Specification1/1 -> EnvTemp/1
  Signal Specification2/1 -> RoadGrade/1
  Vector Concatenate/1 -> WindVel/1
  Signal Specification3/1 -> Vector Concatenate/1  "WindX"
  Constant3/1 -> Signal Specification4/1
  Constant4/1 -> Signal Specification5/1
  Signal Specification4/1 -> Vector Concatenate/2  "WindY"
  Signal Specification5/1 -> Vector Concatenate/3  "WindZ"

== system CAVE_MachE_dSPACE_250912/Vehicle Under Test2/Environment/Subsystem1 ==
  EnvPrs : Inport
  EnvTemp : Inport  Port=2
  WindVel : Inport  Port=3
  RoadGrade : Inport  Port=4
  GroundBus : Inport  Port=5
  Bus Creator : BusCreator  Inputs=5
  Env : Outport
  wires:
  EnvPrs/1 -> Bus Creator/1  "EnvPrs"
  EnvTemp/1 -> Bus Creator/2  "EnvTemp"
  Bus Creator/1 -> Env/1  "Env"
  WindVel/1 -> Bus Creator/3  "WindVel"
  RoadGrade/1 -> Bus Creator/4  "RoadGrade"
  GroundBus/1 -> Bus Creator/5  "GndBus"

== system CAVE_MachE_dSPACE_250912/Vehicle Under Test2/Monitor/Calculate Fuel MPG ==
  Monitor : Inport
  Bus Selector : BusSelector  OutputSignals=Veh.Chassis.VehDist,Veh.Batt.EngPlant.FuellMassFlw
  Constant : Constant  Value=FuelSpecificGrav
  Density of Water : Gain  Gain=997
  Divide : Product  Inputs=*/
  Divide1 : Product  Inputs=*/
  Integrator : Integrator
  Saturation : Saturate  UpperLimit=inf  LowerLimit=1e-7
  Signal Specification : SignalSpecification  Unit=mi
  Signal Specification1 : SignalSpecification  Unit=m^3
  Signal Specification2 : SignalSpecification  Unit=gal
  Unit Conversion : UnitConversion
  Unit Conversion1 : UnitConversion
  FuelEconMPG : Outport
  wires:
  Divide1/1 -> FuelEconMPG/1  "FuelEconMPG"
  Divide/1 -> Signal Specification1/1
  Unit Conversion1/1 -> Signal Specification2/1
  Signal Specification2/1 -> Saturation/1
  Unit Conversion/1 -> Signal Specification/1
  Bus Selector/1 -> Unit Conversion/1  "<VehDist>"
  Bus Selector/2 -> Integrator/1  "<FuellMassFlw>"
  Integrator/1 -> Divide/1  "FuelMass"
  Density of Water/1 -> Divide/2
  Saturation/1 -> Divide1/2  "FuelVolume"
  Constant/1 -> Density of Water/1
  Signal Specification1/1 -> Unit Conversion1/1
  Monitor/1 -> Bus Selector/1
  Signal Specification/1 -> Divide1/1  "VehDistMiles"

== system CAVE_MachE_dSPACE_250912/Vehicle Under Test2/Monitor/Calculate Powertrain Energy ==
  Monitor : Inport
  Bus Selector2 : BusSelector  OutputSignals=Veh.Diff.PwrInfo.PwrTrnsfrd.PwrTrnsfrd.PwrDriveshft
  Integrator : Integrator
  Signal Specification : SignalSpecification  Unit=J
  Signal Specification1 : SignalSpecification  Unit=kW*h
  Unit Conversion : UnitConversion
  TransEnrgyOutkWh : Outport
  wires:
  Unit Conversion/1 -> Signal Specification1/1
  Integrator/1 -> Signal Specification/1  "EnrgyTrans"
  Signal Specification/1 -> Unit Conversion/1
  Signal Specification1/1 -> TransEnrgyOutkWh/1
  Monitor/1 -> Bus Selector2/1
  Bus Selector2/1 -> Integrator/1  "<PwrDriveshft>"

== system CAVE_MachE_dSPACE_250912/Vehicle Under Test2/Vehicle/Actuation and Outputs ==
  note: Driver Commands are [0,100] for both pedal and brake
  Driver Commands : Inport
  CarlaGBS : Inport  Port=2
  APP : Constant  Value=0
  AR_limit : Saturate  UpperLimit=65  LowerLimit=0
  BR_command_0to100 : Constant  Value=0
  BR_limit : Saturate  UpperLimit=70  LowerLimit=0
  Bus Creator : BusCreator  Inputs=2
  Bus Selector1 : BusSelector  OutputSignals=AccelPedalCmd
  Bus Selector3 : BusSelector  OutputSignals=BrakePedalCmd
  Constant : Constant  Value=0
  Constant1 : Constant  Value=0
  Demux : Demux  Outputs=3
  Gain : Gain  Gain=100
  Gain1 : Gain  Gain=100
  MOOG Brake Actuator : Subsystem
  Min threshold for Brake switch : Constant  Value=0
  Multiport Switch1 : MultiPortSwitch  Inputs=4  SaturateOnIntegerOverflow=off  InputSameDT=off
  Multiport Switch2 : MultiPortSwitch  Inputs=4  SaturateOnIntegerOverflow=off  InputSameDT=off
  Pedal Robot Control Selection : Constant  Value=2
  Relational Operator : RelationalOperator  Operator=>  OutDataTypeStr=boolean  InputSameDT=off
  Scope1 : Scope  NumInputPorts=2
  Vehicle Accel Pedal Voltage Output : Subsystem
  bped2br_N : Lookup_n-D  NumberOfTableDimensions=1  BreakpointsForDimension1=[0 0.1 0.2 100]  Table=[0 0 25 100]  InternalRulePriority=Speed  RndMeth=Simplest
  BrakeSwitch : Outport  VectorParamsAs1DForOutWhenUnconnected=off
  CAVE_Driver : Outport  Port=2
  tag scope: BrakeDriver=global, CarlaSteer=global, GasDriver=global
  wires:
  Multiport Switch1/1 -> AR_limit/1
  APP/1 -> Multiport Switch1/2
  Bus Selector1/1 -> Multiport Switch1/3  "<AccelPedalCmd>"
  Multiport Switch2/1 -> BR_limit/1
  Driver Commands/1 -> Bus Selector3/1, Bus Selector1/1
  Pedal Robot Control Selection/1 -> Multiport Switch1/1, Multiport Switch2/1
  BR_command_0to100/1 -> Multiport Switch2/2
  Bus Selector3/1 -> Multiport Switch2/3  "<BrakePedalCmd>"
  bped2br_N/1 -> MOOG Brake Actuator/1(Brake Pedal command [%])
  Min threshold for Brake switch/1 -> Relational Operator/2
  Relational Operator/1 -> BrakeSwitch/1  "BrakeSwitch"
  Constant/1 -> Multiport Switch1/5
  Constant1/1 -> Multiport Switch2/5
  Bus Creator/1 -> CAVE_Driver/1
  AR_limit/1 -> [GasDriver], Bus Creator/1, Vehicle Accel Pedal Voltage Output/1(APP_pct)  "AccelPedalCmd_pct"
  BR_limit/1 -> Bus Creator/2, [BrakeDriver], Relational Operator/1, bped2br_N/1  "BrakePedalCmd_pct"
  Demux/1 -> Gain/1
  Demux/2 -> Gain1/1
  CarlaGBS/1 -> Demux/1
  Gain/1 -> Multiport Switch1/4
  Gain1/1 -> Multiport Switch2/4
  Demux/3 -> [CarlaSteer]
  [GasDriver] -> Scope1/1
  [BrakeDriver] -> Scope1/2

== system CAVE_MachE_dSPACE_250912/Vehicle Under Test2/Vehicle/Battery ==
  Battery : Subsystem
  Subsystem1 : Subsystem
      mask Display: disp('')
  BattOut : PMIOPort  Side=Right
  Batt : Outport
  wires:
  Battery/1(BattSoc) -> Subsystem1/1(BattSoc)
  Battery/2(BattCurr) -> Subsystem1/2(BattCurr)
  Battery/3(BattVolt) -> Subsystem1/3(BattVolt)
  Subsystem1/1(Batt) -> Batt/1
  connections:
  BattOut/RConn1 -- Battery/RConn1

== system CAVE_MachE_dSPACE_250912/Vehicle Under Test2/Vehicle/Driver and Drive Cycle ==
  Veh speed feedback [kph] : Inport
  Veh speed cycle trigger : Inport  Port=2
  SUMO Veh speed Cmd Level : Inport  Port=3
  CarlaRef : Inport  Port=4
  1-D Lookup Table : Lookup_n-D  NumberOfTableDimensions=1  BreakpointsForDimension1=Ref_time  Table=Ref_speed  InternalRulePriority=Speed  RndMeth=Simplest
  Add : Sum
  Add1 : Sum  Inputs=+-
  Add2 : Sum
  Clock : Clock
  Clock1 : Clock
  CoastDown : Lookup_n-D  Commented=on  NumberOfTableDimensions=1  BreakpointsForDimension1=CoastDown.Time  Table=CoastDown.Speed  InternalRulePriority=Speed  RndMeth=Simplest
  Constant : Constant  Value=0
  Data Type Conversion11 : DataTypeConversion  OutDataTypeStr=double  SaturateOnIntegerOverflow=off  RndMeth=Floor  LockScale=on
  Demux : Demux  Outputs=3
  DriveCycleSelect : Constant  Commented=on
  Driver and PI with FF Control : Subsystem
  Gain : Gain  Gain=1/1.609
  Gain1 : Gain  Gain=1/1.609
  Gain2 : Gain  Gain=3.6
  Gain3 : Gain  Gain=3.6
  Get Cycle Clock Time : Subsystem
  MCT : Lookup_n-D  Commented=on  NumberOfTableDimensions=1  BreakpointsForDimension1=MCT.Time  Table=MCT.Speed  InternalRulePriority=Speed  RndMeth=Simplest
  ManSpd : Constant  Value=0
  ManSpdSel1 : Constant  Value=2
  Memory4 : Memory
  Multiport Switch : MultiPortSwitch  Commented=on  Inputs=5  SaturateOnIntegerOverflow=off  InputSameDT=off
  Multiport Switch1 : MultiPortSwitch  Inputs=4  SaturateOnIntegerOverflow=off  InputSameDT=off
  Rate Limiter : RateLimiter  RisingSlewLimit=5  FallingSlewLimit=-5  SampleTimeMode=inherited
  Scope : Scope  NumInputPorts=2
  Switch1 : Switch  Threshold=3  SaturateOnIntegerOverflow=off  InputSameDT=off
  Terminator{,1..3} (4 alike) : Terminator
  Terminator4 : Terminator  Commented=on
  US06 : Lookup_n-D  Commented=on  NumberOfTableDimensions=1  BreakpointsForDimension1=US06.Time  Table=US06.Speed  InternalRulePriority=Speed  RndMeth=Simplest
  US1 : Lookup_n-D  NumberOfTableDimensions=1  BreakpointsForDimension1=US06.Time  Table=US06.Speed  InternalRulePriority=Speed  RndMeth=Simplest
  driver look ahead seconds : Constant  Value=0.5
  limitedMCT : Lookup_n-D  Commented=on  NumberOfTableDimensions=1  BreakpointsForDimension1=limitedMCT.Time  Table=limitedMCT.Speed  InternalRulePriority=Speed  RndMeth=Simplest
  pMCT : Lookup_n-D  Commented=on  NumberOfTableDimensions=1  BreakpointsForDimension1=pMCT.Time  Table=pMCT.Speed  InternalRulePriority=Speed  RndMeth=Simplest
  DriverBus : Outport
  ManSpdSel : Outport  Port=2
  wires:
  Veh speed cycle trigger/1 -> Get Cycle Clock Time/1(Cycle Trigger)
  MCT/1 -> Multiport Switch/5
  US06/1 -> Multiport Switch/4
  Add/1 -> CoastDown/1, pMCT/1, limitedMCT/1, MCT/1, US06/1
  CoastDown/1 -> Multiport Switch/2
  pMCT/1 -> Multiport Switch/3
  DriveCycleSelect/1 -> Multiport Switch/1
  [VehSpdKph] -> Data Type Conversion11/1
  Driver and PI with FF Control/1(DriverBus) -> DriverBus/1
  Data Type Conversion11/1 -> Gain/1, Scope/1, Driver and PI with FF Control/1(Vehicle_Spd_kph)  "Vehicle_Spd_kph"
  Get Cycle Clock Time/1(tCycle) -> Add/2
  driver look ahead seconds/1 -> Add/1
  limitedMCT/1 -> Multiport Switch/6
  Veh speed feedback [kph]/1 -> [VehSpdKph]
  Gain/1 -> Terminator/1  "Vehicle_Spd_mph"
  Gain1/1 -> Terminator1/1  "Vehicle_SpdDmd_mph"
  Multiport Switch1/1 -> Scope/2, Gain1/1, Driver and PI with FF Control/2(Vehicle_SpdDmd_kph)  "RefSpd [km/hr]"
  Rate Limiter/1 -> Multiport Switch1/2
  Multiport Switch/1 -> Terminator4/1
  Gain2/1 -> Multiport Switch1/3
  CarlaRef/1 -> Demux/1
  Demux/1 -> Gain2/1
  Demux/2 -> Terminator2/1
  Demux/3 -> Terminator3/1
  Constant/1 -> Multiport Switch1/5
  Clock1/1 -> US1/1, Add1/1
  ManSpdSel1/1 -> Switch1/2, Multiport Switch1/1, ManSpdSel/1
  1-D Lookup Table/1 -> Add2/1
  Add1/1 -> 1-D Lookup Table/1  "tCycle"
  SUMO Veh speed Cmd Level/1 -> Add2/2
  Switch1/1 -> Add1/2, Memory4/1
  Memory4/1 -> Switch1/1
  Gain3/1 -> Multiport Switch1/4
  Add2/1 -> Gain3/1
  Clock/1 -> Switch1/3
  US1/1 -> Rate Limiter/1

== system CAVE_MachE_dSPACE_250912/Vehicle Under Test2/Vehicle/From CAN ==
  BrakeSwitch : Inport
  Brake switch ource selection : Constant  Value=2
  Bus Creator1 : BusCreator  Inputs=2
  Demux : Demux  Outputs=1
  Ground : Ground
  Ground1 : Ground
  Multiport Switch1 : MultiPortSwitch  Inputs=2  SaturateOnIntegerOverflow=off  InputSameDT=off
  IO_Out : Outport
  wires:
  Bus Creator1/1 -> IO_Out/1  "IO_Out"
  Multiport Switch1/1 -> Bus Creator1/2  "BRAKE_LAMP_BOOL_CAN"
  Demux/1 -> Bus Creator1/1  "STEERING_ANGLE_DEG_CAN"
  Ground/1 -> Demux/1
  Brake switch ource selection/1 -> Multiport Switch1/1
  Ground1/1 -> Multiport Switch1/2  "Brake switch from CAN"
  BrakeSwitch/1 -> Multiport Switch1/3

== system CAVE_MachE_dSPACE_250912/Vehicle Under Test2/Vehicle/Front Wheel Drive ==
  DrvShfTrq : Inport
  Omega : Inport  Port=2
  Ideal Diff : Subsystem  VariantControl=0
  Ideal Diff AWD : Subsystem  VariantControl=Choice
  Real Diff : Subsystem  VariantControl=1
  Diff : Outport  VectorParamsAs1DForOutWhenUnconnected=off
  AxlTrq : Outport  Port=2  VectorParamsAs1DForOutWhenUnconnected=off
  PropShaftSpd : Outport  Port=3  VectorParamsAs1DForOutWhenUnconnected=off
